simulink model "ZRD_seitw_Simulator"  (R2020a)
settings: Solver=VariableStepAuto  StartTime=0.0  StopTime=10.0  RelTol=1e-3
values from neighbouring files (symbols this model uses):
  g = 9.81    [ZRD_laengs.m]    (also in ZRD_laengsbewegung.m; ZRD_seitenbewegung.m)
  Lb = 1    [ZRD_seitenbewegung.m]
  Le = 1    [ZRD_seitenbewegung.m]
  Lp = 1    [ZRD_seitenbewegung.m]
  Lr = 1    [ZRD_seitenbewegung.m]
  Lz = 1    [ZRD_seitenbewegung.m]
  Nb = 1    [ZRD_seitenbewegung.m]
  Nc = 1    [ZRD_seitenbewegung.m]
  Np = 1    [ZRD_seitenbewegung.m]
  Nr = 1    [ZRD_seitenbewegung.m]
  Nz = 0    [ZRD_seitenbewegung.m]
  V0 = 26.9962    [ZRD_laengs.m]    (also in ZRD_laengsbewegung.m = 30; ZRD_seitenbewegung.m = 30)
  Yz = 0    [ZRD_seitenbewegung.m]
settings Model: Creator=Florian  LastModifiedBy=Florian

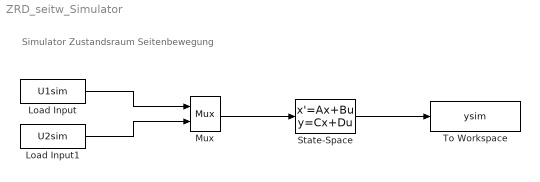
== system ZRD_seitw_Simulator ==
  note: Simulator Zustandsraum Seitenbewegung
  Load Input : FromWorkspace  VariableName=U1sim  SampleTime=-1
  Load Input1 : FromWorkspace  VariableName=U2sim  SampleTime=-1
  Mux : Mux  Inputs=2
  State-Space : StateSpace  A=[Nr, Nb, Np, 0; -1, Yz/V0, 0, g/V0; Lr, Lb, Lp, 0; 0, 0, 1, 0]  B=[Nc, Nz; 0, Yz/V0; Le, Lz; 0, 0]  C=eye(4,4);  D=zeros(4,2)  InitialCondition=zeros(1,4)
  To Workspace : ToWorkspace  VariableName=ysim  SampleTime=-1
  wires:
  Mux/1 -> State-Space/1
  State-Space/1 -> To Workspace/1
  Load Input/1 -> Mux/1
  Load Input1/1 -> Mux/2
